simulink model "Ultrasonic_SFunction"  (R2013a)
settings: Solver=ode45  StartTime=0.0  StopTime=10.0  RelTol=1e-3
settings Model: Creator=carion10  LastModifiedBy=carion10

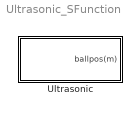
== system Ultrasonic_SFunction ==
  Ultrasonic : Subsystem

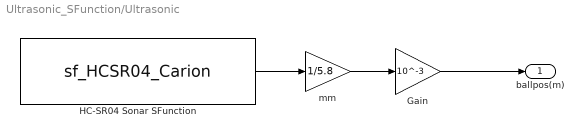
== system Ultrasonic_SFunction/Ultrasonic ==
  Gain : Gain  Gain=10^-3
  HC-SR04 Sonar SFunction : S-Function  InitFcn=try, set_param(gcb,'FunctionName','sf_HCSR04_Carion'), end  FunctionName=sf_HCSR04_Carion  SFunctionModules=sf_HCSR04_Carion_wrapper  EnableBusSupport=off  mask(S-Function Builder){}
      mask help: Simulink:masks:SFunctionBuilder_MD
      mask init:
      | val = [[.9  0.75 0.75 1 1 .9 .9 1]',[1 1 0.75 0.75 .9 .9 1 .9]'];try , sys = get_param(gcb,'SfunBuilderFcnName');if isempty(sys), sys = get_param(gcb,'FunctionName'); end,catch, sys = get_param(gcb,'FunctionName'); end
      settings: CopyFcn=set_param(gcbh,'LinkStatus','none')  PreSaveFcn=try, set_param(gcb,'FunctionName','sf_HCSR04_Carion'), end  OpenFcn=sfunctionwizard(gcbh)
      mask Display: plot(val(:,1),val(:,2)),disp(sys), port_label('output',1,'distance_us')
  mm : Gain  Gain=1/5.8
  ballpos(m) : Outport
  wires:
  HC-SR04 Sonar SFunction/1 -> mm/1
  mm/1 -> Gain/1
  Gain/1 -> ballpos(m)/1
